simulink model "system11"  (R2019a)
settings: Solver=VariableStepAuto  StartTime=0.0  StopTime=10.0  RelTol=1e-3
values from neighbouring files (symbols this model uses):
  b = 0    [Lab2.m]
  d_y0 = 0    [Lab2.m]
  k2 = sqrt(2*k1)    [Lab2.m]    (also in blockFunc10.m)
  y0 = 0    [Lab2.m]
settings Model: Creator=Vasco  LastModifiedBy=Vasco

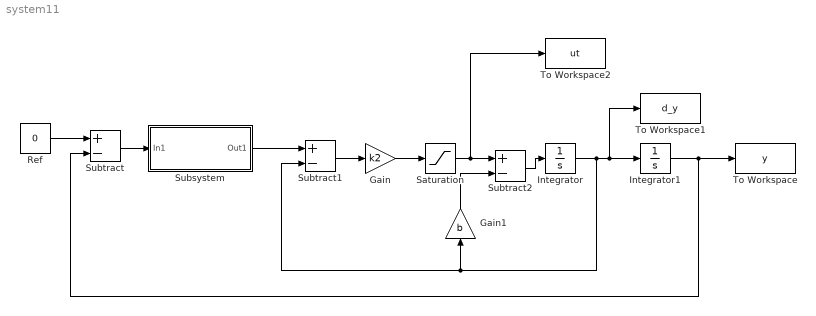
== system system11 ==
  Gain : Gain  Gain=k2
  Gain1 : Gain  Gain=b
  Integrator : Integrator  InitialCondition=d_y0
  Integrator1 : Integrator  InitialCondition=y0
  "Ref " : Constant  Value=0
  Saturation : Saturate  UpperLimit=1  LowerLimit=-1
  Subsystem : Subsystem
  Subtract : Sum  Inputs=+-
  Subtract1 : Sum  Inputs=+-
  Subtract2 : Sum  Inputs=+-
  To Workspace : ToWorkspace  VariableName=y  SampleTime=-1
      settings: Save2DSignal=2-D array (concatenate along first dimension)
  To Workspace1 : ToWorkspace  VariableName=d_y  SampleTime=-1
      settings: Save2DSignal=2-D array (concatenate along first dimension)
  To Workspace2 : ToWorkspace  VariableName=ut  SampleTime=-1
      settings: Save2DSignal=2-D array (concatenate along first dimension)
  wires:
  Integrator1/1 -> To Workspace/1, Subtract/2
  Saturation/1 -> Subtract2/1, To Workspace2/1
  Integrator/1 -> Gain1/1, Subtract1/2, To Workspace1/1, Integrator1/1
  Gain/1 -> Saturation/1
  Subsystem/1(Out1) -> Subtract1/1
  "Ref "/1 -> Subtract/1
  Subtract1/1 -> Gain/1
  Subtract/1 -> Subsystem/1(In1)
  Subtract2/1 -> Integrator/1
  Gain1/1 -> Subtract2/2

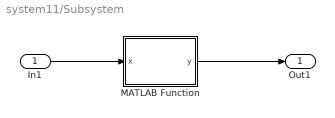
== system system11/Subsystem ==
  In1 : Inport
  MATLAB Function : MATLAB Function  TreatAsAtomicUnit=on
  Out1 : Outport
  wires:
  In1/1 -> MATLAB Function/1(x)
  MATLAB Function/1(y) -> Out1/1

== matlab function system11/Subsystem/MATLAB Function ==
  data: x input; y output
function y = fcn(x)
y1 = 1;
k1 = 1/y1;
k2 = sqrt(2*k1);
    
    if abs(x) <= y1
        y = (k1/k2)*x;
    elseif abs(x) > y1    
        y = sign(x) * (sqrt(2*abs(x))-(1/k2));
    else
        y = 0;
    end

end
